simulink model "torqueWalking"  (Simulink 8.9)
settings: Solver=FixedStepDiscrete  StartTime=0.0  StopTime=Config.t_end  FixedStep=Config.t_step  RelTol=1e-3  EnableMultiTasking=on
InitFcn:
  | cd(fileparts(which(bdroot)));
  | initTorqueWalking;
StopFcn:
  | cd(fileparts(which(bdroot)));
  | outputTorqueWalking
values from neighbouring files (symbols this model uses):
  weights = [1 1 1 1 0.001 0.0001]    [inputWeights.mat]
undefined symbols (not defined in the file or in its folder): biasVectorConstraint_feet, Config, ConstraintMatrix_feet, DiscIntNeverNeededParam, Gains, ROBOT_DOF, Sat
libraries: WBToolboxLibrary x114
(part 4 of 4)

== matlab function Dynamics and Kinematics/Task Accelerations/ComputeTasksPoseAndVelocity/Compose Task Pose and Velocity ==
  data: vel_CoM input double; vel_LFoot input double; vel_RFoot input double; vel_rot_task input double; vel_LHand input double; vel_RHand input double; pos_vel_CoM output double; pose_vel_LFoot output double; pose_vel_RFoot output double; orient_vel_rot_task output double; w_H_CoM input double; w_H_l_sole input double; w_H_r_sole input double; w_H_rot_task input double; w_H_l_hand input double; w_H_r_hand input double; pose_vel_LHand output double; pose_vel_RHand output double
function [pos_vel_CoM, pose_vel_LFoot, pose_vel_RFoot, orient_vel_rot_task, pose_vel_LHand, pose_vel_RHand] = ...
             composeTaskPoseAndVelocityFCN(vel_CoM, vel_LFoot, vel_RFoot, vel_rot_task, vel_LHand, vel_RHand, ...
                                           w_H_CoM, w_H_l_sole, w_H_r_sole, w_H_rot_task, w_H_l_hand, w_H_r_hand)
                                                                                                                              
    [pos_vel_CoM, pose_vel_LFoot, pose_vel_RFoot, orient_vel_rot_task, pose_vel_LHand, pose_vel_RHand] = ...
        composeTaskPoseAndVelocity(vel_CoM, vel_LFoot, vel_RFoot, vel_rot_task, vel_LHand, vel_RHand, ...
                                   w_H_CoM, w_H_l_sole, w_H_r_sole, w_H_rot_task, w_H_l_hand, w_H_r_hand);
end

== matlab function Robot State and References/Gain Scheduling/Gain Scheduling Function ==
  data: state input double; Kp_CoM output double; Kd_CoM output double; Kp_LFoot output double; Kd_LFoot output double; Kp_RFoot output double; Kd_RFoot output double; Kp_rot_task output double; Kd_rot_task output double; Kp_LHand output double; Kd_LHand output double; Kp_RHand output double; Kd_RHand output double; impedances output double; dampings output double; Gains parameter double; smoothingTimeGains output double; Config parameter double
function [Kp_CoM, Kd_CoM, Kp_LFoot, Kd_LFoot, Kp_RFoot, Kd_RFoot, Kp_rot_task, Kd_rot_task, Kp_LHand, Kd_LHand, Kp_RHand, Kd_RHand, impedances, dampings, smoothingTimeGains] = ...
             gainSchedulingFCN(state,Gains,Config)

    [Kp_CoM, Kd_CoM, Kp_LFoot, Kd_LFoot, Kp_RFoot, Kd_RFoot, Kp_rot_task, Kd_rot_task, Kp_LHand, Kd_LHand, Kp_RHand, Kd_RHand, impedances, dampings, smoothingTimeGains] = ...
        gainScheduling(state,Gains,Config);
end

== matlab function Robot State and References/Smooth References /Smooth Reference Orientations/Compute Ref Ang Velocities and Accelerations/Compute Reference Angular Accelerations ==
  data: w_R_LFoot_des input double; w_R_RFoot_des input double; w_R_rot_task_des input double; w_R_LHand_des input double; w_R_RHand_des input double; w_R_LFoot input double; w_R_RFoot input double; omegaDot_LFoot output double; omegaDot_RFoot output double; omegaDot_rot_task output double; w_R_rot_task input double; w_R_LHand input double; w_R_RHand input double; state input double; omega_LFoot input double; omega_RFoot input double; omega_rot_task input double; omega_LHand input double; omega_RHand input double; Config parameter double; omegaDot_LHand output double; omegaDot_RHand output double
function [omegaDot_LFoot, omegaDot_RFoot, omegaDot_rot_task, omegaDot_LHand, omegaDot_RHand] = computeRefAngAccelerationFCN(w_R_LFoot_des, w_R_RFoot_des, w_R_rot_task_des, w_R_LHand_des, w_R_RHand_des, ...
                                                                                            w_R_LFoot, w_R_RFoot, w_R_rot_task, w_R_LHand, w_R_RHand, ...
                                                                                            state, omega_LFoot, omega_RFoot, omega_rot_task, omega_LHand, omega_RHand, Config)
         
    % Compute reference angular accelerations given a desired rotation matrix
    omegaDot_LFoot     = rotationalPID(w_R_LFoot, omega_LFoot, w_R_LFoot_des, zeros(3,1), zeros(3,1), ...
                                       Config.LFoot_Kp_smoothing(state), Config.LFoot_Kd_smoothing(state));
                                   
    omegaDot_RFoot     = rotationalPID(w_R_RFoot, omega_RFoot, w_R_RFoot_des, zeros(3,1), zeros(3,1), ...
                                       Config.RFoot_Kp_smoothing(state), Config.RFoot_Kd_smoothing(state));
                                   
    omegaDot_rot_task  = rotationalPID(w_R_rot_task, omega_rot_task, w_R_rot_task_des, zeros(3,1), zeros(3,1), ...
                                       Config.rot_task_Kp_smoothing(state), Config.rot_task_Kd_smoothing(state));

    omegaDot_LHand     = rotationalPID(w_R_LHand, omega_LHand, w_R_LHand_des, zeros(3,1), zeros(3,1), ...
                                       Config.LHand_Kp_smoothing(state), Config.LHand_Kd_smoothing(state));
                                   
    omegaDot_RHand     = rotationalPID(w_R_RHand, omega_RHand, w_R_RHand_des, zeros(3,1), zeros(3,1), ...
                                       Config.RHand_Kp_smoothing(state), Config.RHand_Kd_smoothing(state));

end

== matlab function Robot State and References/State Machines/Select the Current State and References/STATE MACHINES ==
  data: s_0 input double; w_H_CoM_0 input double; w_H_LFoot_0 input double; w_H_RFoot_0 input double; w_H_rot_task_0 input double; w_H_LHand_0 input double; w_H_RHand_0 input double; LFoot_H_b input double; RFoot_H_b input double; t input double; LFoot_wrench input double; RFoot_wrench input double; state output double; references_CoM output double; references_LFoot output double; references_RFoot output double; references_rot_task output double; references_LHand output double; references_RHand output double; feetInContact output double; references_s output double; w_H_b output double; Config parameter double
function [state, references_CoM, references_LFoot, references_RFoot, references_rot_task, references_LHand, references_RHand, feetInContact, references_s, w_H_b] = stateMachinesFCN ...
             (s_0, w_H_CoM_0, w_H_LFoot_0, w_H_RFoot_0, w_H_rot_task_0, w_H_LHand_0, w_H_RHand_0, LFoot_H_b, RFoot_H_b, ... 
              t, LFoot_wrench, RFoot_wrench, Config)

    [state, references_CoM, references_LFoot, references_RFoot, references_rot_task, references_LHand, references_RHand, feetInContact, references_s, w_H_b] = stateMachineExample ...
        (s_0, w_H_CoM_0, w_H_LFoot_0, w_H_RFoot_0, w_H_rot_task_0, w_H_LHand_0, w_H_RHand_0, t, LFoot_H_b, RFoot_H_b, LFoot_wrench, RFoot_wrench, Config);

end

== matlab function Robot State and References/State Machines/Compute Feet to Base Link Transforms/LFoot to base link transform /fromImuToHomogeousTransformFCN ==
  data: imu_H_link input double; imu_H_link_0 input double; link_H_base input double; inertial_0 input double; inertial input double; neck_pos input double; w_H_b output double; Config parameter double
function w_H_b = worldToBaseTransformWithIMUFCN(imu_H_link,imu_H_link_0,link_H_base,inertial_0,inertial,neck_pos,Config)

    w_H_b = worldToBaseTransformWithIMU(imu_H_link,imu_H_link_0,link_H_base,inertial_0,inertial,neck_pos,Config);

end

== matlab function Robot State and References/Smooth References /Smooth Reference Orientations/Compute Smoothed Ref Orientations/Compute Rotation Matrix Derivative ==
  data: RDot_LFoot output double; RDot_RFoot output double; RDot_rot_task output double; omega_LFoot input double; omega_RFoot input double; omega_rot_task input double; omega_LHand input double; omega_RHand input double; w_R_LFoot input double; w_R_RFoot input double; w_R_rot_task input double; w_R_LHand input double; w_R_RHand input double; RDot_LHand output double; RDot_RHand output double
function [RDot_LFoot, RDot_RFoot, RDot_rot_task, RDot_LHand, RDot_RHand] = rotationDerivativeFromAngVelFCN(omega_LFoot, omega_RFoot, omega_rot_task, omega_LHand, omega_RHand, ... 
                                                                                   w_R_LFoot, w_R_RFoot, w_R_rot_task, w_R_LHand, w_R_RHand)
         
    % Compute the rotation matrix derivative given the angular velocity
    RDot_LFoot     = rotationDerivativeFromAngVel(omega_LFoot,w_R_LFoot);
    RDot_RFoot     = rotationDerivativeFromAngVel(omega_RFoot,w_R_RFoot);
    RDot_rot_task  = rotationDerivativeFromAngVel(omega_rot_task, w_R_rot_task); 
    RDot_LHand     = rotationDerivativeFromAngVel(omega_LHand,w_R_LHand);
    RDot_RHand     = rotationDerivativeFromAngVel(omega_RHand,w_R_RHand);
end

== matlab function Robot State and References/State Machines/Compute Feet to Base Link Transforms/RFoot to base link transform/fromImuToHomogeousTransformFCN ==
  data: imu_H_link input double; imu_H_link_0 input double; link_H_base input double; inertial_0 input double; inertial input double; neck_pos input double; w_H_b output double; Config parameter double
function w_H_b = worldToBaseTransformWithIMUFCN(imu_H_link,imu_H_link_0,link_H_base,inertial_0,inertial,neck_pos,Config)

    w_H_b = worldToBaseTransformWithIMU(imu_H_link,imu_H_link_0,link_H_base,inertial_0,inertial,neck_pos,Config);

end

== matlab function Robot State and References/State Machines/Compute State Velocity/Compute Base Velocity ==
  data: J_LeftFoot input double; J_RightFoot input double; feetInContact input double; nu_b output double; sDot input double; Sat parameter double
function nu_b = computeBaseVelocityFCN(J_LeftFoot, J_RightFoot, feetInContact, sDot, Sat)

    nu_b = computeBaseVelocity(J_LeftFoot, J_RightFoot, feetInContact, sDot, Sat);
end

== matlab function Dynamics and Kinematics/Inverse Kinematics/QP-Based Inverse Kinematics/inverse kinematics integration/Rewrite Base Pose as transformation matrix ==
  data: pose_b input double; w_H_b output double
function  w_H_b = fromPosQuatToTransfMatrFCN(pose_b) 

    % converts the base pose from a position + quaternion representation 
    % to a tranformation matrix
    w_H_b = fromPosQuatToTransfMatr(pose_b);
end

== matlab function Dynamics and Kinematics/Inverse Kinematics/QP-Based Inverse Kinematics/inverse kinematics integration/Compute Base Pose Derivative ==
  data: pose_b input double; nu_b input double; pose_bDot output double
function pose_bDot = basePoseDerivativeFCN(pose_b,nu_b)

    % time derivative of the floating base pose
    pose_bDot = basePoseDerivative(nu_b, pose_b);
end

== matlab function Robot State and References/Smooth References /Smooth Reference Positions/Configure Settling Times ==
  data: state input double; Config parameter double; smoothingTime_CoM output double; smoothingTime_LFoot output double; smoothingTime_RFoot output double; smoothingTime_joints output double; smoothingTime_LHand output double; smoothingTime_RHand output double
function [smoothingTime_CoM, smoothingTime_LFoot, smoothingTime_RFoot, smoothingTime_joints, smoothingTime_LHand, smoothingTime_RHand] = setSmoothingTimesFCN(state,Config)

    [smoothingTime_CoM, smoothingTime_LFoot, smoothingTime_RFoot, smoothingTime_joints, smoothingTime_LHand, smoothingTime_RHand] = setSmoothingTimes(state,Config);

end

== matlab function Dynamics and Kinematics/Inverse Kinematics/QP-Based Inverse Kinematics/inverse kinematics integration/Rewrite Base Pose as pos+quat ==
  data: w_H_b_0 input double; pose_b_0 output double
function pose_b_0 = fromTransfMatrixToPosQuatFCN(w_H_b_0)

    % converts the floating base pose expressed in terms of transformation
    % matrix into position + quaternion representation 
    pose_b_0 = fromTransfMatrixToPosQuat(w_H_b_0);

end

== matlab function Visualization/Cartesian Tasks/MATLAB Function ==
  data: CoM_error input double; errors output double; lFoot_error input double; rFoot_error input double; rotTask_rotError input double; lFoot_rotError input double; rFoot_rotError input double
function errors  = fcn(CoM_error, lFoot_error, rFoot_error, rotTask_rotError, lFoot_rotError, rFoot_rotError)

% cartesian_errors = [norm(CoM_error);
%           norm(lFoot_error);
%           norm(rFoot_error)];
%       
% rotational_errors = [rotTask_rotError;
%                      lFoot_rotError;
%                      rFoot_rotError];
    
errors = [norm(CoM_error)  ;
          rotTask_rotError ;
          norm(lFoot_error);
          lFoot_rotError   ;
          norm(rFoot_error);
          rFoot_rotError  ];

== matlab function Dynamics and Kinematics/Compute Dynamic and Kinematic Quantities/Mass Matrix and Bias Forces/Add motors reflected inertias/Add motor reflected inertias ==
  data: M input double; M_with_inertia output double; Config parameter double
function M_with_inertia = addMotorsInertiaFCN(M,Config)

    M_with_inertia = addMotorsInertia(M,Config);

end

== matlab function Visualization/MATLAB Function ==
  data: joint_errors input double; joint_error_norm output double; tau_measured input double; tau_norm output double; exitFlagQP input double; exitFlagQP_norm output double
function [joint_error_norm, tau_norm, exitFlagQP_norm]  = fcn(joint_errors, tau_measured, exitFlagQP)

joint_error_norm = norm(joint_errors);
tau_norm = norm(tau_measured);
exitFlagQP_norm = norm(exitFlagQP);

== matlab function Visualization/ZMPs/MATLAB Function ==
  data: fz_left input double; fz_right input double; Lcop input double; zmp output double; Rcop input double; pose_lFoot input double; orient_lFoot input double; pose_rFoot input double; orient_rFoot input double; feetInContact input double
function zmp = fcn(fz_left, fz_right,Lcop,Rcop, pose_lFoot, orient_lFoot, pose_rFoot, orient_rFoot, feetInContact)
%#codegen ,Lcontact,Rcontact,

if feetInContact(1) > 0.1 && feetInContact(2) > 0.1 %Both feet on ground
    Lcop        = orient_lFoot(1:2,1:2)*Lcop + pose_lFoot(1:2); %Lcontact(1:2,1:2)*Lcop + Lcontact(1:2,4);
    Rcop        = orient_rFoot(1:2,1:2)*Rcop + pose_rFoot(1:2); %Rcontact(1:2,1:2)*Rcop + Rcontact(1:2,4);
    zmp         = (fz_left*Lcop + fz_right*Rcop)/(fz_left+fz_right);
    
elseif feetInContact(1) > 0.1 %Left foot on ground
    Lcop        = orient_lFoot(1:2,1:2)*Lcop + pose_lFoot(1:2); %Lcontact(1:2,1:2)*Lcop + Lcontact(1:2,4);
    zmp         = (fz_left*Lcop)/(fz_left);
    
elseif feetInContact(2) > 0.1 %Right foot on ground
    Rcop        = orient_rFoot(1:2,1:2)*Rcop + pose_rFoot(1:2); %Rcontact(1:2,1:2)*Rcop + Rcontact(1:2,4);
    zmp         = (fz_right*Rcop)/(fz_right);
    
else
    zmp = zeros(2,1);
end
